simulink model "HANcoder_E407_TTA_Controller_v3"  (R2018b)
settings: Solver=FixedStepDiscrete  StartTime=0.0  StopTime=1  FixedStep=0.01  RelTol=1e-3
PreLoadFcn:
  | librarySetup
  | eval([bdroot,'_startup']) %Calling [modelName]_startup.m
values from neighbouring files (symbols this model uses):
  basic_cycle_duration_bc0 = TM_Reset_Board   + COMP_duration    (= 212)    [HANcoder_E407_TTA_Controller_v3_startup.m]
  basic_cycle_duration_bc1 = TM_Reset_Var_bc1 + COMP_duration    (= 288)    [HANcoder_E407_TTA_Controller_v3_startup.m]
  comm_delay_estimation1 = round(comm_delay_measured1*hardware_granularity/frequency_IRQ)    [HANcoder_E407_TTA_Controller_v3_startup.m]
  comm_delay_estimation2 = round(comm_delay_measured2*hardware_granularity/frequency_IRQ)    [HANcoder_E407_TTA_Controller_v3_startup.m]
  COMM_Period = 40    [HANcoder_E407_TTA_Controller_v3_startup.m]
  COMM_Phase1 = 5    [HANcoder_E407_TTA_Controller_v3_startup.m]
  COMM_Phase2 = 8    [HANcoder_E407_TTA_Controller_v3_startup.m]
  COMP_duration = 4    [HANcoder_E407_TTA_Controller_v3_startup.m]
  Controller1_Board = 1    [HANcoder_E407_TTA_Controller_v3_startup.m]
  Controller2_Board = 2    [HANcoder_E407_TTA_Controller_v3_startup.m]
  Controller3_Board = 3    [HANcoder_E407_TTA_Controller_v3_startup.m]
  delta_a_set = Simulink.Parameter    [HANcoder_E407_TTA_Controller_v3_startup.m]
  delta_f_set = Simulink.Parameter    [HANcoder_E407_TTA_Controller_v3_startup.m]
  delta_max = 1    [HANcoder_E407_TTA_Controller_v3_startup.m]
  delta_min = -1    [HANcoder_E407_TTA_Controller_v3_startup.m]
  delta_precision = 6    [HANcoder_E407_TTA_Controller_v3_startup.m]
  e_width = 0.1    [HANcoder_E407_TTA_Controller_v3_startup.m]
  frequency_IRQ = 100    [HANcoder_E407_TTA_Controller_v3_startup.m]
  HANtuneOverride = Simulink.Parameter    [HANcoder_E407_TTA_Controller_v3_startup.m]
  hardware_granularity = 1000000    [HANcoder_E407_TTA_Controller_v3_startup.m]
  I_a = 2.25    [HANcoder_E407_TTA_Controller_v3_startup.m]
  I_f = 2.25    [HANcoder_E407_TTA_Controller_v3_startup.m]
  idle_time_init = basic_cycle_duration_bc0 + basic_cycle_duration_bc1    (= 500)    [HANcoder_E407_TTA_Controller_v3_startup.m]
  Input_Gen_Board = 4    [HANcoder_E407_TTA_Controller_v3_startup.m]
  LA_Clock_Gr = 1    [HANcoder_E407_TTA_Controller_v3_startup.m]
  LA_COMM_dly = 0    [HANcoder_E407_TTA_Controller_v3_startup.m]
  LA_COMM_Err = 0    [HANcoder_E407_TTA_Controller_v3_startup.m]
  LA_E_Desync = 0    [HANcoder_E407_TTA_Controller_v3_startup.m]
  LA_MEX_Flag = 1    [HANcoder_E407_TTA_Controller_v3_startup.m]
  LA_Task_Act = 1    [HANcoder_E407_TTA_Controller_v3_startup.m]
  m_v = 100.0    (= 100)    [HANcoder_E407_TTA_Controller_v3_startup.m]
  Master_Role = 1    [HANcoder_E407_TTA_Controller_v3_startup.m]
  matrix_cycle_duration = basic_cycle_duration_bc0 + basic_cycle_duration_bc1    (= 500)    [HANcoder_E407_TTA_Controller_v3_startup.m]
  matrix_rows = 2    [HANcoder_E407_TTA_Controller_v3_startup.m]
  max_num_msgs_CAN1 = 2^Tx_bit_number-1    (= 7)    [HANcoder_E407_TTA_Controller_v3_startup.m]
  max_num_msgs_CAN2 = max_num_msgs_CAN1    (= 7)    [HANcoder_E407_TTA_Controller_v3_startup.m]
  OutControl1_ID = 23    [HANcoder_E407_TTA_Controller_v3_startup.m]
  OutControl2_ID = 24    [HANcoder_E407_TTA_Controller_v3_startup.m]
  OutEmulator_ID = 25    [HANcoder_E407_TTA_Controller_v3_startup.m]
  R_al = 0.10    (= 0.1)    [HANcoder_E407_TTA_Controller_v3_startup.m]
  R_ar = 0.10    (= 0.1)    [HANcoder_E407_TTA_Controller_v3_startup.m]
  R_fl = 0.10    (= 0.1)    [HANcoder_E407_TTA_Controller_v3_startup.m]
  R_fr = 0.10    (= 0.1)    [HANcoder_E407_TTA_Controller_v3_startup.m]
  script_run = Simulink.Parameter    [HANcoder_E407_TTA_Controller_v3_startup.m]
  SensorValues_ID = 22    [HANcoder_E407_TTA_Controller_v3_startup.m]
  SetValues_ID = 21    [HANcoder_E407_TTA_Controller_v3_startup.m]
  Slave_Role = 2    [HANcoder_E407_TTA_Controller_v3_startup.m]
  speed_k_d = Simulink.Parameter    [HANcoder_E407_TTA_Controller_v3_startup.m]
  speed_k_i = Simulink.Parameter    [HANcoder_E407_TTA_Controller_v3_startup.m]
  speed_k_p = Simulink.Parameter    [HANcoder_E407_TTA_Controller_v3_startup.m]
  speed_max = 10    [HANcoder_E407_TTA_Controller_v3_startup.m]
  speed_min = -10    [HANcoder_E407_TTA_Controller_v3_startup.m]
  speed_precision = 3    [HANcoder_E407_TTA_Controller_v3_startup.m]
  Sync_ID = 1    [HANcoder_E407_TTA_Controller_v3_startup.m]
  tau_max = 5    [HANcoder_E407_TTA_Controller_v3_startup.m]
  tau_min = -5    [HANcoder_E407_TTA_Controller_v3_startup.m]
  tau_range = abs(tau_max) + abs(tau_min)    [HANcoder_E407_TTA_Controller_v3_startup.m]
  theta_max = (speed_max/R_fr)*matrix_cycle_duration*frequency_IRQ/hardware_granularity    (= 5)    [HANcoder_E407_TTA_Controller_v3_startup.m]
  theta_min = (-1)*theta_max    (= -5)    [HANcoder_E407_TTA_Controller_v3_startup.m]
  theta_precision = 7-(fix(log2(theta_max))+1)    [HANcoder_E407_TTA_Controller_v3_startup.m]
  Tl_a = 0.6    [HANcoder_E407_TTA_Controller_v3_startup.m]
  Tl_f = 0.6    [HANcoder_E407_TTA_Controller_v3_startup.m]
  TM_Check_Output_Control1 = TM_COMM_Output_Control1 + COMM_duration    (= 188)    [HANcoder_E407_TTA_Controller_v3_startup.m]
  TM_Check_Output_Control2 = TM_COMM_Output_Control2 + COMM_duration    (= 232)    [HANcoder_E407_TTA_Controller_v3_startup.m]
  TM_Check_Output_Emulator = TM_COMM_Output_Emulator + COMM_duration    (= 280)    [HANcoder_E407_TTA_Controller_v3_startup.m]
  TM_Check_Sensor_Values = TM_COMM_Sensor_Values + COMM_duration    (= 132)    [HANcoder_E407_TTA_Controller_v3_startup.m]
  TM_Check_Set_Values = TM_COMM_Set_Values + COMM_duration    (= 88)    [HANcoder_E407_TTA_Controller_v3_startup.m]
  TM_Check_Sync = TM_COMM_Sync   + COMM_duration    (= 40)    [HANcoder_E407_TTA_Controller_v3_startup.m]
  TM_Check_TOuts = TM_Count_Vote3 + COMP_duration    (= 196)    [HANcoder_E407_TTA_Controller_v3_startup.m]
  TM_Check_Vote1 = TM_COMM_Vote1  + COMM_duration    (= 92)    [HANcoder_E407_TTA_Controller_v3_startup.m]
  TM_Check_Vote2 = TM_COMM_Vote2  + COMM_duration    (= 140)    [HANcoder_E407_TTA_Controller_v3_startup.m]
  TM_Check_Vote3 = TM_COMM_Vote3  + COMM_duration    (= 188)    [HANcoder_E407_TTA_Controller_v3_startup.m]
  TM_COMM_Output_Control1 = TM_Velocity + COMP_duration    (= 148)    [HANcoder_E407_TTA_Controller_v3_startup.m]
  TM_COMM_Output_Control2 = TM_Check_Output_Control1 + COMP_duration    (= 192)    [HANcoder_E407_TTA_Controller_v3_startup.m]
  TM_COMM_Output_Emulator = TM_TMR + COMP_duration    (= 240)    [HANcoder_E407_TTA_Controller_v3_startup.m]
  TM_COMM_Sensor_Values = TM_Check_Set_Values + COMP_duration    (= 92)    [HANcoder_E407_TTA_Controller_v3_startup.m]
  TM_COMM_Set_Values = TM_Update_LT + COMP_duration    (= 48)    [HANcoder_E407_TTA_Controller_v3_startup.m]
  TM_COMM_Sync = basic_cycle_start    (= 0)    [HANcoder_E407_TTA_Controller_v3_startup.m]
  TM_COMM_Vote1 = TM_Vote_Dec    + COMP_duration    (= 52)    [HANcoder_E407_TTA_Controller_v3_startup.m]
  TM_COMM_Vote2 = TM_Count_Vote1 + COMP_duration    (= 100)    [HANcoder_E407_TTA_Controller_v3_startup.m]
  TM_COMM_Vote3 = TM_Count_Vote2 + COMP_duration    (= 148)    [HANcoder_E407_TTA_Controller_v3_startup.m]
  TM_Count_Vote1 = TM_Check_Vote1 + COMP_duration    (= 96)    [HANcoder_E407_TTA_Controller_v3_startup.m]
  TM_Count_Vote2 = TM_Check_Vote2 + COMP_duration    (= 144)    [HANcoder_E407_TTA_Controller_v3_startup.m]
  TM_Count_Vote3 = TM_Check_Vote3 + COMP_duration    (= 192)    [HANcoder_E407_TTA_Controller_v3_startup.m]
  TM_Data_bc0 = TM_COMM_Sync    (= 0)    [HANcoder_E407_TTA_Controller_v3_startup.m]
  TM_Data_bc1 = TM_Data_bc0(1:3)    [HANcoder_E407_TTA_Controller_v3_startup.m]
  TM_New_Master = TM_Check_TOuts + COMP_duration    (= 200)    [HANcoder_E407_TTA_Controller_v3_startup.m]
  TM_Reset_Board = TM_Reset_Var   + COMP_duration    (= 208)    [HANcoder_E407_TTA_Controller_v3_startup.m]
  TM_Reset_Var = TM_New_Master  + COMP_duration    (= 204)    [HANcoder_E407_TTA_Controller_v3_startup.m]
  TM_Reset_Var_bc1 = TM_Check_Output_Emulator + COMP_duration    (= 284)    [HANcoder_E407_TTA_Controller_v3_startup.m]
  TM_Steer = TM_Check_Sensor_Values + COMP_duration    (= 136)    [HANcoder_E407_TTA_Controller_v3_startup.m]
  TM_TMR = TM_Check_Output_Control2 + COMP_duration    (= 236)    [HANcoder_E407_TTA_Controller_v3_startup.m]
  TM_Torque = TM_Steer + COMP_duration    (= 140)    [HANcoder_E407_TTA_Controller_v3_startup.m]
  TM_Type_bc0 = COMM    (= 0)    [HANcoder_E407_TTA_Controller_v3_startup.m]
  TM_Type_bc1 = TM_Type_bc0(1:3)    [HANcoder_E407_TTA_Controller_v3_startup.m]
  TM_Update_LT = TM_Check_Sync  + COMP_duration    (= 44)    [HANcoder_E407_TTA_Controller_v3_startup.m]
  TM_Velocity = TM_Torque + COMP_duration    (= 144)    [HANcoder_E407_TTA_Controller_v3_startup.m]
  TM_Vote_Dec = TM_Update_LT   + COMP_duration    (= 48)    [HANcoder_E407_TTA_Controller_v3_startup.m]
  torque_a_k_d = Simulink.Parameter    [HANcoder_E407_TTA_Controller_v3_startup.m]
  torque_a_k_i = Simulink.Parameter    [HANcoder_E407_TTA_Controller_v3_startup.m]
  torque_a_k_p = Simulink.Parameter    [HANcoder_E407_TTA_Controller_v3_startup.m]
  torque_f_k_d = Simulink.Parameter    [HANcoder_E407_TTA_Controller_v3_startup.m]
  torque_f_k_i = Simulink.Parameter    [HANcoder_E407_TTA_Controller_v3_startup.m]
  torque_f_k_p = Simulink.Parameter    [HANcoder_E407_TTA_Controller_v3_startup.m]
  torque_precision = 4    [HANcoder_E407_TTA_Controller_v3_startup.m]
  v_set = Simulink.Parameter    [HANcoder_E407_TTA_Controller_v3_startup.m]
  Vehicle_Em_Board = 5    [HANcoder_E407_TTA_Controller_v3_startup.m]
  Vote1_ID = 11    [HANcoder_E407_TTA_Controller_v3_startup.m]
  Vote2_ID = 12    [HANcoder_E407_TTA_Controller_v3_startup.m]
  Vote3_ID = 13    [HANcoder_E407_TTA_Controller_v3_startup.m]
undefined symbols (not defined in the file or in its folder): A0, A1, A2, A3, A4, CON2, CON4, D10, D12, D13, D8, D9
libraries: hdlsllib x352, HANcoder_STM32_Target x28, simulink x3, simulink_extras x1
(part 22 of 33)

== system HANcoder_E407_TTA_Controller_v3/HANcoder STM32 Target - E407-STM32 algorithm/Global Ticks Increment/CAN Management/Matrix Cycle Manager/Input Generator Matrix Cycle/input generator basic cycle 1/COMM Task - Set_Values/Reception substasks/RX buffers update ==
  note: Reset RX Buffer Flag
  note: Reception ID
      |    Sync Msg: 1
      |    Vote Node 1: 11
      |    Vote Node 2: 12
      |    Vote Node 3: 13
  note: Wait until new message
      | arrives
  note: Reset RX Buffer Flag
  note: Reception ID
      |    Sync Msg: 1
      |    Vote Node 1: 11
      |    Vote Node 2: 12
      |    Vote Node 3: 13
  note: Wait until new message
      | arrives
  note: Reset Rx buffers
  note: Reception end - Set RxID and Reset CAN buffer flags
  note: CAN1
  note: CAN2
  Rx_ID : Inport
  Enable : EnablePort
  Cast13 : DataTypeConversion  OutDataTypeStr=uint32
  Cast14 : DataTypeConversion  OutDataTypeStr=boolean
  Cast15 : DataTypeConversion  OutDataTypeStr=uint8
  Cast3 : DataTypeConversion  OutDataTypeStr=uint32
  Cast5 : DataTypeConversion  OutDataTypeStr=boolean
  Cast6 : DataTypeConversion  OutDataTypeStr=uint8
  Data Store Write : DataStoreWrite  DataStoreName=Msg_Rx
  Data Store Write11 : DataStoreWrite  DataStoreName=RxID_CAN2
  Data Store Write12 : DataStoreWrite  DataStoreName=Rx_State_CAN2
  Data Store Write2 : DataStoreWrite  DataStoreName=New_Msg_Ready_CAN1
  Data Store Write3 : DataStoreWrite  DataStoreName=new_msg_Rx
  Data Store Write6 : DataStoreWrite  DataStoreName=RxID_CAN1
  Data Store Write7 : DataStoreWrite  DataStoreName=Rx_State_CAN1
  Data Store Write9 : DataStoreWrite  DataStoreName=New_Msg_Ready_CAN2
  RESET1 : Constant  Value=0
  RESET2 : Constant  Value=0
  RESET_CAN1_new_buffer : Constant  Value=0
  RESET_CAN2_new_buffer : Constant  Value=0
  RESET_Msg_Rx : Constant  Value=0  OutDataTypeStr=Bus: msg_buffer_type
  RESET_new_msg_Rx : Constant  Value=0  OutDataTypeStr=boolean
  wires:
  Cast13/1 -> Data Store Write11/1
  Rx_ID/1 -> Cast3/1, Cast13/1
  RESET2/1 -> Cast14/1
  Cast14/1 -> Data Store Write9/1
  RESET_CAN2_new_buffer/1 -> Cast15/1
  Cast15/1 -> Data Store Write12/1
  Cast6/1 -> Data Store Write7/1
  RESET_CAN1_new_buffer/1 -> Cast6/1
  RESET_new_msg_Rx/1 -> Data Store Write3/1
  RESET_Msg_Rx/1 -> Data Store Write/1
  Cast5/1 -> Data Store Write2/1
  RESET1/1 -> Cast5/1
  Cast3/1 -> Data Store Write6/1

== system HANcoder_E407_TTA_Controller_v3/HANcoder STM32 Target - E407-STM32 algorithm/Global Ticks Increment/CAN Management/Matrix Cycle Manager/Input Generator Matrix Cycle/input generator basic cycle 1/COMM Task - Set_Values/Transmission subtasks/Check msg transmission CAN1 ==
  note: The TX buffers are updated one tick
      | before the message is sent
  note: A message should be sent during
      | this tick through CAN1
  note: In the next tick, a message will be
      | sent through CAN1
  Local Time : Inport
  Time Mark : Inport  Port=2
  Tx_ID : Inport  Port=3
  Value Domain Msg : Inport  Port=4
  Enable : EnablePort
  Constant11 : Constant  Value=0
  Constant22 : Constant
  Constant24 : Constant  Value=COMM_Phase1
  Constant27 : Constant  Value=COMM_Phase1
  Constant8 : Constant  Value=0
  Equal4 : RelationalOperator  Operator===  OutDataTypeStr=boolean  RndMeth=Simplest
  Equal7 : RelationalOperator  Operator===  OutDataTypeStr=boolean  RndMeth=Simplest
  Minus : Sum  Inputs=++-
  Minus1 : Sum  Inputs=+-
  Mod : Math  Operator=mod  SaturateOnIntegerOverflow=on
  Mod1 : Math  Operator=mod  SaturateOnIntegerOverflow=on
  TX buffer update CAN1 : Subsystem  Priority=20
  Send CAN1 : Outport  OutputWhenDisabled=reset  InitialOutput=0
  wires:
  Time Mark/1 -> Minus1/2, Minus/3
  Equal4/1 -> TX buffer update CAN1/Enable
  Constant22/1 -> Minus/2
  Local Time/1 -> Minus1/1, Minus/1
  Tx_ID/1 -> TX buffer update CAN1/1(Tx_ID)
  Mod1/1 -> Equal7/1
  Constant27/1 -> Mod1/2
  Minus/1 -> Mod/1
  Value Domain Msg/1 -> TX buffer update CAN1/2(Msg_Value_Data)
  Constant24/1 -> Mod/2
  Mod/1 -> Equal4/1
  Minus1/1 -> Mod1/1
  Constant11/1 -> Equal7/2
  Equal7/1 -> Send CAN1/1
  Constant8/1 -> Equal4/2

== system HANcoder_E407_TTA_Controller_v3/HANcoder STM32 Target - E407-STM32 algorithm/Global Ticks Increment/CAN Management/Matrix Cycle Manager/Input Generator Matrix Cycle/input generator basic cycle 1/COMM Task - Set_Values/Transmission subtasks/Check msg transmission CAN2 ==
  note: In the next tick, a message will be
      | sent through CAN2
  note: A message should be sent during
      | this tick through CAN2
  note: The TX buffers are updated one tick
      | before the message is sent
  Local Time : Inport
  Time Mark : Inport  Port=2
  Tx_ID : Inport  Port=3
  Value Domain Msg : Inport  Port=4
  Enable : EnablePort
  Constant11 : Constant  Value=0
  Constant22 : Constant
  Constant24 : Constant  Value=COMM_Phase2
  Constant27 : Constant  Value=COMM_Phase2
  Constant8 : Constant  Value=0
  Equal4 : RelationalOperator  Operator===  OutDataTypeStr=boolean  RndMeth=Simplest
  Equal7 : RelationalOperator  Operator===  OutDataTypeStr=boolean  RndMeth=Simplest
  Minus : Sum  Inputs=++-
  Minus1 : Sum  Inputs=+-
  Mod : Math  Operator=mod  SaturateOnIntegerOverflow=on
  Mod1 : Math  Operator=mod  SaturateOnIntegerOverflow=on
  TX buffer update CAN2 : Subsystem  Priority=20
  Send CAN2 : Outport  OutputWhenDisabled=reset  InitialOutput=0
  wires:
  Constant8/1 -> Equal4/2
  Equal7/1 -> Send CAN2/1
  Constant11/1 -> Equal7/2
  Minus1/1 -> Mod1/1
  Mod/1 -> Equal4/1
  Constant24/1 -> Mod/2
  Value Domain Msg/1 -> TX buffer update CAN2/2(Msg_Value_Data)
  Minus/1 -> Mod/1
  Constant27/1 -> Mod1/2
  Mod1/1 -> Equal7/1
  Tx_ID/1 -> TX buffer update CAN2/1(Tx_ID)
  Local Time/1 -> Minus/1, Minus1/1
  Constant22/1 -> Minus/2
  Equal4/1 -> TX buffer update CAN2/Enable
  Time Mark/1 -> Minus/3, Minus1/2

== system HANcoder_E407_TTA_Controller_v3/HANcoder STM32 Target - E407-STM32 algorithm/Global Ticks Increment/CAN Management/Matrix Cycle Manager/Input Generator Matrix Cycle/input generator basic cycle 1/COMM Task - Set_Values/Transmission subtasks/Msg_Value_Data_Encoded5 ==
  note: Value domain message encoding
      | <Warning!> The first buffer (from the top) is not used in transmission!
  Enable : EnablePort
  Bus Creator : BusCreator  Inputs=8  OutDataTypeStr=Bus: msg_buffer_type
  Constant : Constant  Value=0  OutDataTypeStr=uint8
  Constant1 : Constant  Value=delta_precision
  Constant10 : Constant  Value=delta_f_set
  Constant11 : Constant  Value=delta_a_set
  Constant12 : Constant  Value=v_set
  Constant2 : Constant  Value=delta_precision
  Constant3 : Constant  Value=speed_precision
  Constant4 : Constant  Value=delta_max
  Constant5 : Constant  Value=delta_min
  Constant6 : Constant  Value=delta_max
  Constant7 : Constant  Value=delta_min
  Constant8 : Constant  Value=speed_max
  Constant9 : Constant  Value=speed_min
  float2uint1 : Subsystem
  float2uint2 : Subsystem
  float2uint8 : Subsystem
  Value_domain_msg : Outport
  wires:
  Constant9/1 -> float2uint2/4(magnitude_min)
  Constant8/1 -> float2uint2/3(magnitude_max)
  Constant12/1 -> float2uint2/2(magnitude)
  Constant3/1 -> float2uint2/1(precision)
  Constant7/1 -> float2uint1/4(magnitude_min)
  Constant6/1 -> float2uint1/3(magnitude_max)
  Constant11/1 -> float2uint1/2(magnitude)
  Constant2/1 -> float2uint1/1(precision)
  Constant1/1 -> float2uint8/1(precision)
  Constant10/1 -> float2uint8/2(magnitude)
  Constant4/1 -> float2uint8/3(magnitude_max)
  Constant5/1 -> float2uint8/4(magnitude_min)
  float2uint2/1(coded) -> Bus Creator/4
  float2uint1/1(coded) -> Bus Creator/3
  float2uint8/1(coded) -> Bus Creator/2
  Constant/1 -> Bus Creator/6, Bus Creator/8, Bus Creator/7, Bus Creator/5, Bus Creator/1
  Bus Creator/1 -> Value_domain_msg/1

== system HANcoder_E407_TTA_Controller_v3/HANcoder STM32 Target - E407-STM32 algorithm/Global Ticks Increment/CAN Management/Matrix Cycle Manager/Input Generator Matrix Cycle/input generator basic cycle 1/COMM Task - Sync bc 1/Reception substasks/RX buffers update ==
  note: CAN2
  note: CAN1
  note: Reception end - Set RxID and Reset CAN buffer flags
  note: Reset Rx buffers
  note: Wait until new message
      | arrives
  note: Reception ID
      |    Sync Msg: 1
      |    Vote Node 1: 11
      |    Vote Node 2: 12
      |    Vote Node 3: 13
  note: Reset RX Buffer Flag
  note: Wait until new message
      | arrives
  note: Reception ID
      |    Sync Msg: 1
      |    Vote Node 1: 11
      |    Vote Node 2: 12
      |    Vote Node 3: 13
  note: Reset RX Buffer Flag
  Rx_ID : Inport
  Enable : EnablePort
  Cast13 : DataTypeConversion  OutDataTypeStr=uint32
  Cast14 : DataTypeConversion  OutDataTypeStr=boolean
  Cast15 : DataTypeConversion  OutDataTypeStr=uint8
  Cast3 : DataTypeConversion  OutDataTypeStr=uint32
  Cast5 : DataTypeConversion  OutDataTypeStr=boolean
  Cast6 : DataTypeConversion  OutDataTypeStr=uint8
  Data Store Write : DataStoreWrite  DataStoreName=Msg_Rx
  Data Store Write11 : DataStoreWrite  DataStoreName=RxID_CAN2
  Data Store Write12 : DataStoreWrite  DataStoreName=Rx_State_CAN2
  Data Store Write2 : DataStoreWrite  DataStoreName=New_Msg_Ready_CAN1
  Data Store Write3 : DataStoreWrite  DataStoreName=new_msg_Rx
  Data Store Write6 : DataStoreWrite  DataStoreName=RxID_CAN1
  Data Store Write7 : DataStoreWrite  DataStoreName=Rx_State_CAN1
  Data Store Write9 : DataStoreWrite  DataStoreName=New_Msg_Ready_CAN2
  RESET1 : Constant  Value=0
  RESET2 : Constant  Value=0
  RESET_CAN1_new_buffer : Constant  Value=0
  RESET_CAN2_new_buffer : Constant  Value=0
  RESET_Msg_Rx : Constant  Value=0  OutDataTypeStr=Bus: msg_buffer_type
  RESET_new_msg_Rx : Constant  Value=0  OutDataTypeStr=boolean
  wires:
  Cast3/1 -> Data Store Write6/1
  RESET1/1 -> Cast5/1
  Cast5/1 -> Data Store Write2/1
  RESET_Msg_Rx/1 -> Data Store Write/1
  RESET_new_msg_Rx/1 -> Data Store Write3/1
  RESET_CAN1_new_buffer/1 -> Cast6/1
  Cast6/1 -> Data Store Write7/1
  Cast15/1 -> Data Store Write12/1
  RESET_CAN2_new_buffer/1 -> Cast15/1
  Cast14/1 -> Data Store Write9/1
  RESET2/1 -> Cast14/1
  Rx_ID/1 -> Cast13/1, Cast3/1
  Cast13/1 -> Data Store Write11/1

== system HANcoder_E407_TTA_Controller_v3/HANcoder STM32 Target - E407-STM32 algorithm/Global Ticks Increment/CAN Management/Matrix Cycle Manager/Input Generator Matrix Cycle/input generator basic cycle 1/COMM Task - Sync bc 1/Transmission subtasks/Check msg transmission CAN1 ==
  note: In the next tick, a message will be
      | sent through CAN1
  note: A message should be sent during
      | this tick through CAN1
  note: The TX buffers are updated one tick
      | before the message is sent
  Local Time : Inport
  Time Mark : Inport  Port=2
  Tx_ID : Inport  Port=3
  Value Domain Msg : Inport  Port=4
  Enable : EnablePort
  Constant11 : Constant  Value=0
  Constant22 : Constant
  Constant24 : Constant  Value=COMM_Phase1
  Constant27 : Constant  Value=COMM_Phase1
  Constant8 : Constant  Value=0
  Equal4 : RelationalOperator  Operator===  OutDataTypeStr=boolean  RndMeth=Simplest
  Equal7 : RelationalOperator  Operator===  OutDataTypeStr=boolean  RndMeth=Simplest
  Minus : Sum  Inputs=++-
  Minus1 : Sum  Inputs=+-
  Mod : Math  Operator=mod  SaturateOnIntegerOverflow=on
  Mod1 : Math  Operator=mod  SaturateOnIntegerOverflow=on
  TX buffer update CAN1 : Subsystem  Priority=20
  Send CAN1 : Outport  OutputWhenDisabled=reset  InitialOutput=0
  wires:
  Constant8/1 -> Equal4/2
  Equal7/1 -> Send CAN1/1
  Constant11/1 -> Equal7/2
  Minus1/1 -> Mod1/1
  Mod/1 -> Equal4/1
  Constant24/1 -> Mod/2
  Value Domain Msg/1 -> TX buffer update CAN1/2(Msg_Value_Data)
  Minus/1 -> Mod/1
  Constant27/1 -> Mod1/2
  Mod1/1 -> Equal7/1
  Tx_ID/1 -> TX buffer update CAN1/1(Tx_ID)
  Local Time/1 -> Minus/1, Minus1/1
  Constant22/1 -> Minus/2
  Equal4/1 -> TX buffer update CAN1/Enable
  Time Mark/1 -> Minus/3, Minus1/2

== system HANcoder_E407_TTA_Controller_v3/HANcoder STM32 Target - E407-STM32 algorithm/Global Ticks Increment/CAN Management/Matrix Cycle Manager/Input Generator Matrix Cycle/input generator basic cycle 1/COMM Task - Sync bc 1/Transmission subtasks/Check msg transmission CAN2 ==
  note: The TX buffers are updated one tick
      | before the message is sent
  note: A message should be sent during
      | this tick through CAN2
  note: In the next tick, a message will be
      | sent through CAN2
  Local Time : Inport
  Time Mark : Inport  Port=2
  Tx_ID : Inport  Port=3
  Value Domain Msg : Inport  Port=4
  Enable : EnablePort
  Constant11 : Constant  Value=0
  Constant22 : Constant
  Constant24 : Constant  Value=COMM_Phase2
  Constant27 : Constant  Value=COMM_Phase2
  Constant8 : Constant  Value=0
  Equal4 : RelationalOperator  Operator===  OutDataTypeStr=boolean  RndMeth=Simplest
  Equal7 : RelationalOperator  Operator===  OutDataTypeStr=boolean  RndMeth=Simplest
  Minus : Sum  Inputs=++-
  Minus1 : Sum  Inputs=+-
  Mod : Math  Operator=mod  SaturateOnIntegerOverflow=on
  Mod1 : Math  Operator=mod  SaturateOnIntegerOverflow=on
  TX buffer update CAN2 : Subsystem  Priority=20
  Send CAN2 : Outport  OutputWhenDisabled=reset  InitialOutput=0
  wires:
  Time Mark/1 -> Minus1/2, Minus/3
  Equal4/1 -> TX buffer update CAN2/Enable
  Constant22/1 -> Minus/2
  Local Time/1 -> Minus1/1, Minus/1
  Tx_ID/1 -> TX buffer update CAN2/1(Tx_ID)
  Mod1/1 -> Equal7/1
  Constant27/1 -> Mod1/2
  Minus/1 -> Mod/1
  Value Domain Msg/1 -> TX buffer update CAN2/2(Msg_Value_Data)
  Constant24/1 -> Mod/2
  Mod/1 -> Equal4/1
  Minus1/1 -> Mod1/1
  Constant11/1 -> Equal7/2
  Equal7/1 -> Send CAN2/1
  Constant8/1 -> Equal4/2

== system HANcoder_E407_TTA_Controller_v3/HANcoder STM32 Target - E407-STM32 algorithm/Global Ticks Increment/CAN Management/Matrix Cycle Manager/Input Generator Matrix Cycle/input generator basic cycle 1/COMM Task - Sync bc 1/Transmission subtasks/Msg_Value_Data_Encoded ==
  note: Value domain message encoding
      | <Warning!> The first buffer (from the top) is not used in transmission!
  Enable : EnablePort
  Bus Creator : BusCreator  Inputs=8  OutDataTypeStr=Bus: msg_buffer_type
  Constant : Constant  Value=0  OutDataTypeStr=uint8
  Constant1 : Constant  Value=torque_precision
  Constant10 : Constant  Value=speed_max
  Constant11 : Constant  Value=speed_min
  Constant12 : Constant  Value=delta_max
  Constant13 : Constant  Value=delta_min
  Constant14 : Constant  Value=delta_max
  Constant15 : Constant  Value=delta_min
  Constant2 : Constant  Value=torque_precision
  Constant3 : Constant  Value=speed_precision
  Constant4 : Constant  Value=delta_precision
  Constant5 : Constant  Value=delta_precision
  Constant6 : Constant  Value=tau_max
  Constant7 : Constant  Value=tau_min
  Constant8 : Constant  Value=tau_max
  Constant9 : Constant  Value=tau_min
  Data Store Read33 : DataStoreRead  DataStoreName=speed_integral
  Data Store Read34 : DataStoreRead  DataStoreName=torque_ar_integral
  Data Store Read35 : DataStoreRead  DataStoreName=torque_fr_integral
  Data Store Read36 : DataStoreRead  DataStoreName=delta_a_est
  Data Store Read37 : DataStoreRead  DataStoreName=delta_f_est
  float2uint1 : Subsystem
  float2uint2 : Subsystem
  float2uint3 : Subsystem
  float2uint4 : Subsystem
  float2uint8 : Subsystem
  Value_domain_msg : Outport
  wires:
  Constant15/1 -> float2uint4/4(magnitude_min)
  Constant14/1 -> float2uint4/3(magnitude_max)
  Constant12/1 -> float2uint3/3(magnitude_max)
  Constant13/1 -> float2uint3/4(magnitude_min)
  Constant11/1 -> float2uint2/4(magnitude_min)
  Constant10/1 -> float2uint2/3(magnitude_max)
  Constant8/1 -> float2uint1/3(magnitude_max)
  Constant9/1 -> float2uint1/4(magnitude_min)
  Constant7/1 -> float2uint8/4(magnitude_min)
  Constant6/1 -> float2uint8/3(magnitude_max)
  float2uint4/1(coded) -> Bus Creator/6
  float2uint3/1(coded) -> Bus Creator/5
  float2uint2/1(coded) -> Bus Creator/4
  float2uint1/1(coded) -> Bus Creator/3
  float2uint8/1(coded) -> Bus Creator/2
  Data Store Read36/1 -> float2uint4/2(magnitude)
  Data Store Read37/1 -> float2uint3/2(magnitude)
  Data Store Read33/1 -> float2uint2/2(magnitude)
  Data Store Read34/1 -> float2uint1/2(magnitude)
  Data Store Read35/1 -> float2uint8/2(magnitude)
  Constant/1 -> Bus Creator/7, Bus Creator/8, Bus Creator/1
  Constant5/1 -> float2uint4/1(precision)
  Constant4/1 -> float2uint3/1(precision)
  Constant3/1 -> float2uint2/1(precision)
  Constant2/1 -> float2uint1/1(precision)
  Constant1/1 -> float2uint8/1(precision)
  Bus Creator/1 -> Value_domain_msg/1

== system HANcoder_E407_TTA_Controller_v3/HANcoder STM32 Target - E407-STM32 algorithm/Global Ticks Increment/CAN Management/Matrix Cycle Manager/Input Generator Matrix Cycle/input generator basic cycle 1/COMP Task - Sync bc1 check/Process_Messages/Demux message CAN1 and check coherence ==
  CAN1_Rx_msg : Inport  OutDataTypeStr=Bus: msg_buffer_type
  expected_basic_cycle : Inport  Port=2
  Enable : EnablePort
  Bus Creator : BusCreator  Inputs=8  OutDataTypeStr=Bus: msg_buffer_type
  Bus Selector : BusSelector  OutputSignals=Buffer_1,Buffer_2,Buffer_3,Buffer_4,Buffer_5,Buffer_6,Buffer_7,Buffer_8
  Constant : Constant  Value=0  OutDataTypeStr=uint8
  Equal1 : RelationalOperator  Operator===  OutDataTypeStr=boolean  RndMeth=Simplest
  Subsystem : Subsystem
  Terminator : Terminator
  msg_count>2_DEBUG : Subsystem
  CAN1_msg : Outport  OutDataTypeStr=Bus: msg_buffer_type
  Msg_Count_CAN1 : Outport  Port=2
  CAN1_msg_coherent : Outport  Port=3  OutputWhenDisabled=reset  InitialOutput=0
  wires:
  Constant/1 -> Bus Creator/1
  Bus Creator/1 -> CAN1_msg/1
  Subsystem/2(msg_count) -> Msg_Count_CAN1/1, msg_count>2_DEBUG/1(msg_c)
  Subsystem/1(basic_cycle) -> Equal1/1
  Bus Selector/1 -> Subsystem/1(Msg_Temporal_Data)  "<Buffer_1>"
  Bus Selector/4 -> Bus Creator/4  "<Buffer_4>"
  Bus Selector/8 -> Bus Creator/8  "<Buffer_8>"
  Bus Selector/7 -> Bus Creator/7  "<Buffer_7>"
  Bus Selector/5 -> Bus Creator/5  "<Buffer_5>"
  Bus Selector/6 -> Bus Creator/6  "<Buffer_6>"
  expected_basic_cycle/1 -> Equal1/2
  Equal1/1 -> CAN1_msg_coherent/1
  CAN1_Rx_msg/1 -> Bus Selector/1
  Bus Selector/3 -> Bus Creator/3  "<Buffer_3>"
  Bus Selector/2 -> Bus Creator/2  "<Buffer_2>"
  Subsystem/3(board_id) -> Terminator/1

== system HANcoder_E407_TTA_Controller_v3/HANcoder STM32 Target - E407-STM32 algorithm/Global Ticks Increment/CAN Management/Matrix Cycle Manager/Input Generator Matrix Cycle/input generator basic cycle 1/COMP Task - Sync bc1 check/Process_Messages/Demux message CAN1 and check coherence1 ==
  CAN2_Rx_msg : Inport  OutDataTypeStr=Bus: msg_buffer_type
  expected_basic_cycle : Inport  Port=2
  Enable : EnablePort
  Bus Creator : BusCreator  Inputs=8  OutDataTypeStr=Bus: msg_buffer_type
  Bus Selector : BusSelector  OutputSignals=Buffer_1,Buffer_2,Buffer_3,Buffer_4,Buffer_5,Buffer_6,Buffer_7,Buffer_8
  Constant : Constant  Value=0  OutDataTypeStr=uint8
  Equal1 : RelationalOperator  Operator===  OutDataTypeStr=boolean  RndMeth=Simplest
  Subsystem : Subsystem
  Terminator : Terminator
  msg_count>2_DEBUG : Subsystem
  CAN2_msg_coherent : Outport  OutputWhenDisabled=reset  InitialOutput=0
  Msg_Count_CAN2 : Outport  Port=2
  CAN2_msg : Outport  Port=3  OutDataTypeStr=Bus: msg_buffer_type
  wires:
  Constant/1 -> Bus Creator/1
  Bus Creator/1 -> CAN2_msg/1
  Subsystem/2(msg_count) -> Msg_Count_CAN2/1, msg_count>2_DEBUG/1(msg_c)
  Subsystem/1(basic_cycle) -> Equal1/1
  Bus Selector/1 -> Subsystem/1(Msg_Temporal_Data)  "<Buffer_1>"
  Bus Selector/4 -> Bus Creator/4  "<Buffer_4>"
  Bus Selector/8 -> Bus Creator/8  "<Buffer_8>"
  Bus Selector/7 -> Bus Creator/7  "<Buffer_7>"
  Bus Selector/5 -> Bus Creator/5  "<Buffer_5>"
  Bus Selector/6 -> Bus Creator/6  "<Buffer_6>"
  expected_basic_cycle/1 -> Equal1/2
  Equal1/1 -> CAN2_msg_coherent/1
  CAN2_Rx_msg/1 -> Bus Selector/1
  Bus Selector/3 -> Bus Creator/3  "<Buffer_3>"
  Bus Selector/2 -> Bus Creator/2  "<Buffer_2>"
  Subsystem/3(board_id) -> Terminator/1

== system HANcoder_E407_TTA_Controller_v3/HANcoder STM32 Target - E407-STM32 algorithm/Global Ticks Increment/CAN Management/Matrix Cycle Manager/Input Generator Matrix Cycle/input generator basic cycle 1/COMP Task - Sync bc1 check/Process_Messages/Desync calculation ==
  note: Estimation of the Local Time when the message was sent
  note: Desync CAN2
      | expected RX - Actual RX
  note: Desync CAN1
      | expected RX - Actual RX
  TM_COMM : Inport
  New_msg_CAN1 : Inport  Port=2
  msg_count_CAN1 : Inport  Port=3
  msg_count_CAN2 : Inport  Port=4
  Enable : EnablePort
  Constant : Constant  Value=COMM_Phase1
  Constant1 : Constant  Value=COMM_Phase2
  Data Store Read : DataStoreRead  DataStoreName=Msg_Rx_Ticks_CAN1
  Data Store Read1 : DataStoreRead  DataStoreName=Msg_Rx_Ticks_CAN2
  Data Store Write1 : DataStoreWrite  Priority=23  DataStoreName=Desync_Ticks
  Minus : Sum  Priority=21  Inputs=+-
  Minus1 : Sum  Priority=20  Inputs=+-
  Multiply : Product  Priority=10
  Multiply1 : Product  Priority=12
  Sum : Sum  Priority=11  Inputs=+++
  Sum1 : Sum  Priority=13  Inputs=+++
  Switch1 : Switch  Priority=22  Criteria=u2 > Threshold
  delay_estimation_1 : Constant  Value=comm_delay_estimation1
  delay_estimation_2 : Constant  Value=comm_delay_estimation2
  wires:
  TM_COMM/1 -> Sum1/2, Sum/2
  delay_estimation_1/1 -> Sum/3
  msg_count_CAN1/1 -> Multiply/2
  Switch1/1 -> Data Store Write1/1  "Desync_Sync_bc1_ing_s"
  Minus/1 -> Switch1/3
  Sum1/1 -> [expected_LT_CAN2]
  delay_estimation_2/1 -> Sum1/3
  Multiply1/1 -> Sum1/1
  [expected_LT_CAN1] -> Minus1/1
  [expected_LT_CAN2] -> Minus/1
  Data Store Read1/1 -> Minus/2
  Multiply/1 -> Sum/1
  Data Store Read/1 -> Minus1/2
  msg_count_CAN2/1 -> Multiply1/2
  Sum/1 -> [expected_LT_CAN1]
  Minus1/1 -> Switch1/1
  Constant/1 -> Multiply/1
  Constant1/1 -> Multiply1/1
  New_msg_CAN1/1 -> Switch1/2

== system HANcoder_E407_TTA_Controller_v3/HANcoder STM32 Target - E407-STM32 algorithm/Global Ticks Increment/CAN Management/Matrix Cycle Manager/Input Generator Matrix Cycle/input generator basic cycle 1/COMP Task - Update LT/Local Time Update/Desync_Negative ==
  note: Local Time Update
  note: Current Local Time correction
  note: Local time correction when Desync is negative
      | In this case the Local Time "goes back in time".
      | Previous tasks will not be activated because
      | sync_processed flag is alread set.
  Current_Local_Time : Inport
  Enable : EnablePort
  Cast : DataTypeConversion  Priority=13  OutDataTypeStr=uint16
  Data Store Read : DataStoreRead  Priority=11  DataStoreName=Desync_Ticks
  Data Store Write1 : DataStoreWrite  Priority=14  DataStoreName=Local_Ticks  DataStoreElements=Local_Ticks
  Minus : Sum  Priority=12
  wires:
  Current_Local_Time/1 -> Minus/1
  Cast/1 -> Data Store Write1/1
  Minus/1 -> Cast/1
  Data Store Read/1 -> Minus/2

== system HANcoder_E407_TTA_Controller_v3/HANcoder STM32 Target - E407-STM32 algorithm/Global Ticks Increment/CAN Management/Matrix Cycle Manager/Vehicle Emulator Matrix Cycle/vehicle emulator basic cycle 0/COMM Task - Sync bc 0/Reception substasks/RX buffers update ==
  note: Reset RX Buffer Flag
  note: Reception ID
      |    Sync Msg: 1
      |    Vote Node 1: 11
      |    Vote Node 2: 12
      |    Vote Node 3: 13
  note: Wait until new message
      | arrives
  note: Reset RX Buffer Flag
  note: Reception ID
      |    Sync Msg: 1
      |    Vote Node 1: 11
      |    Vote Node 2: 12
      |    Vote Node 3: 13
  note: Wait until new message
      | arrives
  note: Reset Rx buffers
  note: Reception end - Set RxID and Reset CAN buffer flags
  note: CAN1
  note: CAN2
  Rx_ID : Inport
  Enable : EnablePort
  Cast13 : DataTypeConversion  OutDataTypeStr=uint32
  Cast14 : DataTypeConversion  OutDataTypeStr=boolean
  Cast15 : DataTypeConversion  OutDataTypeStr=uint8
  Cast3 : DataTypeConversion  OutDataTypeStr=uint32
  Cast5 : DataTypeConversion  OutDataTypeStr=boolean
  Cast6 : DataTypeConversion  OutDataTypeStr=uint8
  Data Store Write : DataStoreWrite  DataStoreName=Msg_Rx
  Data Store Write11 : DataStoreWrite  DataStoreName=RxID_CAN2
  Data Store Write12 : DataStoreWrite  DataStoreName=Rx_State_CAN2
  Data Store Write2 : DataStoreWrite  DataStoreName=New_Msg_Ready_CAN1
  Data Store Write3 : DataStoreWrite  DataStoreName=new_msg_Rx
  Data Store Write6 : DataStoreWrite  DataStoreName=RxID_CAN1
  Data Store Write7 : DataStoreWrite  DataStoreName=Rx_State_CAN1
  Data Store Write9 : DataStoreWrite  DataStoreName=New_Msg_Ready_CAN2
  RESET1 : Constant  Value=0
  RESET2 : Constant  Value=0
  RESET_CAN1_new_buffer : Constant  Value=0
  RESET_CAN2_new_buffer : Constant  Value=0
  RESET_Msg_Rx : Constant  Value=0  OutDataTypeStr=Bus: msg_buffer_type
  RESET_new_msg_Rx : Constant  Value=0  OutDataTypeStr=boolean
  wires:
  Cast13/1 -> Data Store Write11/1
  Rx_ID/1 -> Cast3/1, Cast13/1
  RESET2/1 -> Cast14/1
  Cast14/1 -> Data Store Write9/1
  RESET_CAN2_new_buffer/1 -> Cast15/1
  Cast15/1 -> Data Store Write12/1
  Cast6/1 -> Data Store Write7/1
  RESET_CAN1_new_buffer/1 -> Cast6/1
  RESET_new_msg_Rx/1 -> Data Store Write3/1
  RESET_Msg_Rx/1 -> Data Store Write/1
  Cast5/1 -> Data Store Write2/1
  RESET1/1 -> Cast5/1
  Cast3/1 -> Data Store Write6/1

== system HANcoder_E407_TTA_Controller_v3/HANcoder STM32 Target - E407-STM32 algorithm/Global Ticks Increment/CAN Management/Matrix Cycle Manager/Vehicle Emulator Matrix Cycle/vehicle emulator basic cycle 0/COMM Task - Sync bc 0/Transmission subtasks/Check msg transmission CAN1 ==
  note: The TX buffers are updated one tick
      | before the message is sent
  note: A message should be sent during
      | this tick through CAN1
  note: In the next tick, a message will be
      | sent through CAN1
  Local Time : Inport
  Time Mark : Inport  Port=2
  Tx_ID : Inport  Port=3
  Value Domain Msg : Inport  Port=4
  Enable : EnablePort
  Constant11 : Constant  Value=0
  Constant22 : Constant
  Constant24 : Constant  Value=COMM_Phase1
  Constant27 : Constant  Value=COMM_Phase1
  Constant8 : Constant  Value=0
  Equal4 : RelationalOperator  Operator===  OutDataTypeStr=boolean  RndMeth=Simplest
  Equal7 : RelationalOperator  Operator===  OutDataTypeStr=boolean  RndMeth=Simplest
  Minus : Sum  Inputs=++-
  Minus1 : Sum  Inputs=+-
  Mod : Math  Operator=mod  SaturateOnIntegerOverflow=on
  Mod1 : Math  Operator=mod  SaturateOnIntegerOverflow=on
  TX buffer update CAN1 : Subsystem  Priority=20
  Send CAN1 : Outport  OutputWhenDisabled=reset  InitialOutput=0
  wires:
  Time Mark/1 -> Minus1/2, Minus/3
  Equal4/1 -> TX buffer update CAN1/Enable
  Constant22/1 -> Minus/2
  Local Time/1 -> Minus1/1, Minus/1
  Tx_ID/1 -> TX buffer update CAN1/1(Tx_ID)
  Mod1/1 -> Equal7/1
  Constant27/1 -> Mod1/2
  Minus/1 -> Mod/1
  Value Domain Msg/1 -> TX buffer update CAN1/2(Msg_Value_Data)
  Constant24/1 -> Mod/2
  Mod/1 -> Equal4/1
  Minus1/1 -> Mod1/1
  Constant11/1 -> Equal7/2
  Equal7/1 -> Send CAN1/1
  Constant8/1 -> Equal4/2

== system HANcoder_E407_TTA_Controller_v3/HANcoder STM32 Target - E407-STM32 algorithm/Global Ticks Increment/CAN Management/Matrix Cycle Manager/Vehicle Emulator Matrix Cycle/vehicle emulator basic cycle 0/COMM Task - Sync bc 0/Transmission subtasks/Check msg transmission CAN2 ==
  note: In the next tick, a message will be
      | sent through CAN2
  note: A message should be sent during
      | this tick through CAN2
  note: The TX buffers are updated one tick
      | before the message is sent
  Local Time : Inport
  Time Mark : Inport  Port=2
  Tx_ID : Inport  Port=3
  Value Domain Msg : Inport  Port=4
  Enable : EnablePort
  Constant11 : Constant  Value=0
  Constant22 : Constant
  Constant24 : Constant  Value=COMM_Phase2
  Constant27 : Constant  Value=COMM_Phase2
  Constant8 : Constant  Value=0
  Equal4 : RelationalOperator  Operator===  OutDataTypeStr=boolean  RndMeth=Simplest
  Equal7 : RelationalOperator  Operator===  OutDataTypeStr=boolean  RndMeth=Simplest
  Minus : Sum  Inputs=++-
  Minus1 : Sum  Inputs=+-
  Mod : Math  Operator=mod  SaturateOnIntegerOverflow=on
  Mod1 : Math  Operator=mod  SaturateOnIntegerOverflow=on
  TX buffer update CAN2 : Subsystem  Priority=20
  Send CAN2 : Outport  OutputWhenDisabled=reset  InitialOutput=0
  wires:
  Constant8/1 -> Equal4/2
  Equal7/1 -> Send CAN2/1
  Constant11/1 -> Equal7/2
  Minus1/1 -> Mod1/1
  Mod/1 -> Equal4/1
  Constant24/1 -> Mod/2
  Value Domain Msg/1 -> TX buffer update CAN2/2(Msg_Value_Data)
  Minus/1 -> Mod/1
  Constant27/1 -> Mod1/2
  Mod1/1 -> Equal7/1
  Tx_ID/1 -> TX buffer update CAN2/1(Tx_ID)
  Local Time/1 -> Minus/1, Minus1/1
  Constant22/1 -> Minus/2
  Equal4/1 -> TX buffer update CAN2/Enable
  Time Mark/1 -> Minus/3, Minus1/2

== system HANcoder_E407_TTA_Controller_v3/HANcoder STM32 Target - E407-STM32 algorithm/Global Ticks Increment/CAN Management/Matrix Cycle Manager/Vehicle Emulator Matrix Cycle/vehicle emulator basic cycle 0/COMM Task - Sync bc 0/Transmission subtasks/Msg_Value_Data_Encoded ==
  note: Value domain message encoding
      | <Warning!> The first buffer (from the top) is not used in transmission!
  Enable : EnablePort
  Bus Creator : BusCreator  Inputs=8  OutDataTypeStr=Bus: msg_buffer_type
  Constant : Constant  Value=0  OutDataTypeStr=uint8
  Constant1 : Constant  Value=torque_precision
  Constant10 : Constant  Value=speed_max
  Constant11 : Constant  Value=speed_min
  Constant12 : Constant  Value=delta_max
  Constant13 : Constant  Value=delta_min
  Constant14 : Constant  Value=delta_max
  Constant15 : Constant  Value=delta_min
  Constant2 : Constant  Value=torque_precision
  Constant3 : Constant  Value=speed_precision
  Constant4 : Constant  Value=delta_precision
  Constant5 : Constant  Value=delta_precision
  Constant6 : Constant  Value=tau_max
  Constant7 : Constant  Value=tau_min
  Constant8 : Constant  Value=tau_max
  Constant9 : Constant  Value=tau_min
  Data Store Read33 : DataStoreRead  DataStoreName=speed_integral
  Data Store Read34 : DataStoreRead  DataStoreName=torque_ar_integral
  Data Store Read35 : DataStoreRead  DataStoreName=torque_fr_integral
  Data Store Read36 : DataStoreRead  DataStoreName=delta_a_est
  Data Store Read37 : DataStoreRead  DataStoreName=delta_f_est
  float2uint1 : Subsystem
  float2uint2 : Subsystem
  float2uint3 : Subsystem
  float2uint4 : Subsystem
  float2uint8 : Subsystem
  Value_domain_msg : Outport
  wires:
  Bus Creator/1 -> Value_domain_msg/1
  Constant1/1 -> float2uint8/1(precision)
  Constant2/1 -> float2uint1/1(precision)
  Constant3/1 -> float2uint2/1(precision)
  Constant4/1 -> float2uint3/1(precision)
  Constant5/1 -> float2uint4/1(precision)
  Constant/1 -> Bus Creator/1, Bus Creator/8, Bus Creator/7
  Data Store Read35/1 -> float2uint8/2(magnitude)
  Data Store Read34/1 -> float2uint1/2(magnitude)
  Data Store Read33/1 -> float2uint2/2(magnitude)
  Data Store Read37/1 -> float2uint3/2(magnitude)
  Data Store Read36/1 -> float2uint4/2(magnitude)
  float2uint8/1(coded) -> Bus Creator/2
  float2uint1/1(coded) -> Bus Creator/3
  float2uint2/1(coded) -> Bus Creator/4
  float2uint3/1(coded) -> Bus Creator/5
  float2uint4/1(coded) -> Bus Creator/6
  Constant6/1 -> float2uint8/3(magnitude_max)
  Constant7/1 -> float2uint8/4(magnitude_min)
  Constant9/1 -> float2uint1/4(magnitude_min)
  Constant8/1 -> float2uint1/3(magnitude_max)
  Constant10/1 -> float2uint2/3(magnitude_max)
  Constant11/1 -> float2uint2/4(magnitude_min)
  Constant13/1 -> float2uint3/4(magnitude_min)
  Constant12/1 -> float2uint3/3(magnitude_max)
  Constant14/1 -> float2uint4/3(magnitude_max)
  Constant15/1 -> float2uint4/4(magnitude_min)

== system HANcoder_E407_TTA_Controller_v3/HANcoder STM32 Target - E407-STM32 algorithm/Global Ticks Increment/CAN Management/Matrix Cycle Manager/Vehicle Emulator Matrix Cycle/vehicle emulator basic cycle 0/COMP Task - Sync bc0 check/Process_Messages/Demux message CAN1 and check coherence ==
  CAN1_Rx_msg : Inport  OutDataTypeStr=Bus: msg_buffer_type
  expected_basic_cycle : Inport  Port=2
  Enable : EnablePort
  Bus Creator : BusCreator  Inputs=8  OutDataTypeStr=Bus: msg_buffer_type
  Bus Selector : BusSelector  OutputSignals=Buffer_1,Buffer_2,Buffer_3,Buffer_4,Buffer_5,Buffer_6,Buffer_7,Buffer_8
  Constant : Constant  Value=0  OutDataTypeStr=uint8
  Equal1 : RelationalOperator  Operator===  OutDataTypeStr=boolean  RndMeth=Simplest
  Subsystem : Subsystem
  Terminator : Terminator
  msg_count>2_DEBUG : Subsystem
  CAN1_msg : Outport  OutDataTypeStr=Bus: msg_buffer_type
  Msg_Count_CAN1 : Outport  Port=2
  CAN1_msg_coherent : Outport  Port=3  OutputWhenDisabled=reset  InitialOutput=0
  wires:
  Bus Selector/2 -> Bus Creator/2  "<Buffer_2>"
  Bus Selector/3 -> Bus Creator/3  "<Buffer_3>"
  CAN1_Rx_msg/1 -> Bus Selector/1
  Equal1/1 -> CAN1_msg_coherent/1
  expected_basic_cycle/1 -> Equal1/2
  Bus Selector/6 -> Bus Creator/6  "<Buffer_6>"
  Bus Selector/5 -> Bus Creator/5  "<Buffer_5>"
  Bus Selector/7 -> Bus Creator/7  "<Buffer_7>"
  Bus Selector/8 -> Bus Creator/8  "<Buffer_8>"
  Bus Selector/4 -> Bus Creator/4  "<Buffer_4>"
  Bus Selector/1 -> Subsystem/1(Msg_Temporal_Data)  "<Buffer_1>"
  Subsystem/1(basic_cycle) -> Equal1/1
  Subsystem/2(msg_count) -> msg_count>2_DEBUG/1(msg_c), Msg_Count_CAN1/1
  Bus Creator/1 -> CAN1_msg/1
  Constant/1 -> Bus Creator/1
  Subsystem/3(board_id) -> Terminator/1

== system HANcoder_E407_TTA_Controller_v3/HANcoder STM32 Target - E407-STM32 algorithm/Global Ticks Increment/CAN Management/Matrix Cycle Manager/Vehicle Emulator Matrix Cycle/vehicle emulator basic cycle 0/COMP Task - Sync bc0 check/Process_Messages/Demux message CAN1 and check coherence1 ==
  CAN2_Rx_msg : Inport  OutDataTypeStr=Bus: msg_buffer_type
  expected_basic_cycle : Inport  Port=2
  Enable : EnablePort
  Bus Creator : BusCreator  Inputs=8  OutDataTypeStr=Bus: msg_buffer_type
  Bus Selector : BusSelector  OutputSignals=Buffer_1,Buffer_2,Buffer_3,Buffer_4,Buffer_5,Buffer_6,Buffer_7,Buffer_8
  Constant : Constant  Value=0  OutDataTypeStr=uint8
  Equal1 : RelationalOperator  Operator===  OutDataTypeStr=boolean  RndMeth=Simplest
  Subsystem : Subsystem
  Terminator : Terminator
  msg_count>2_DEBUG : Subsystem
  CAN2_msg_coherent : Outport  OutputWhenDisabled=reset  InitialOutput=0
  Msg_Count_CAN2 : Outport  Port=2
  CAN2_msg : Outport  Port=3  OutDataTypeStr=Bus: msg_buffer_type
  wires:
  Bus Selector/2 -> Bus Creator/2  "<Buffer_2>"
  Bus Selector/3 -> Bus Creator/3  "<Buffer_3>"
  CAN2_Rx_msg/1 -> Bus Selector/1
  Equal1/1 -> CAN2_msg_coherent/1
  expected_basic_cycle/1 -> Equal1/2
  Bus Selector/6 -> Bus Creator/6  "<Buffer_6>"
  Bus Selector/5 -> Bus Creator/5  "<Buffer_5>"
  Bus Selector/7 -> Bus Creator/7  "<Buffer_7>"
  Bus Selector/8 -> Bus Creator/8  "<Buffer_8>"
  Bus Selector/4 -> Bus Creator/4  "<Buffer_4>"
  Bus Selector/1 -> Subsystem/1(Msg_Temporal_Data)  "<Buffer_1>"
  Subsystem/1(basic_cycle) -> Equal1/1
  Subsystem/2(msg_count) -> msg_count>2_DEBUG/1(msg_c), Msg_Count_CAN2/1
  Bus Creator/1 -> CAN2_msg/1
  Constant/1 -> Bus Creator/1
  Subsystem/3(board_id) -> Terminator/1

== system HANcoder_E407_TTA_Controller_v3/HANcoder STM32 Target - E407-STM32 algorithm/Global Ticks Increment/CAN Management/Matrix Cycle Manager/Vehicle Emulator Matrix Cycle/vehicle emulator basic cycle 0/COMP Task - Sync bc0 check/Process_Messages/Desync calculation ==
  note: Estimation of the Local Time when the message was sent
  note: Desync CAN2
      | expected RX - Actual RX
  note: Desync CAN1
      | expected RX - Actual RX
  TM_COMM : Inport
  New_msg_CAN1 : Inport  Port=2
  msg_count_CAN1 : Inport  Port=3
  msg_count_CAN2 : Inport  Port=4
  Enable : EnablePort
  Constant : Constant  Value=COMM_Phase1
  Constant1 : Constant  Value=COMM_Phase2
  Data Store Read : DataStoreRead  DataStoreName=Msg_Rx_Ticks_CAN1
  Data Store Read1 : DataStoreRead  DataStoreName=Msg_Rx_Ticks_CAN2
  Data Store Write1 : DataStoreWrite  Priority=23  DataStoreName=Desync_Ticks
  Minus : Sum  Priority=21  Inputs=+-
  Minus1 : Sum  Priority=20  Inputs=+-
  Multiply : Product  Priority=10
  Multiply1 : Product  Priority=12
  Sum : Sum  Priority=11  Inputs=+++
  Sum1 : Sum  Priority=13  Inputs=+++
  Switch1 : Switch  Priority=22  Criteria=u2 > Threshold
  delay_estimation_1 : Constant  Value=comm_delay_estimation1
  delay_estimation_2 : Constant  Value=comm_delay_estimation2
  wires:
  TM_COMM/1 -> Sum1/2, Sum/2
  delay_estimation_1/1 -> Sum/3
  msg_count_CAN1/1 -> Multiply/2
  Switch1/1 -> Data Store Write1/1  "Desync_Sync_bc0_vem_s"
  Minus/1 -> Switch1/3
  Sum1/1 -> [expected_LT_CAN2]
  delay_estimation_2/1 -> Sum1/3
  Multiply1/1 -> Sum1/1
  [expected_LT_CAN1] -> Minus1/1
  [expected_LT_CAN2] -> Minus/1
  Data Store Read1/1 -> Minus/2
  Multiply/1 -> Sum/1
  Data Store Read/1 -> Minus1/2
  msg_count_CAN2/1 -> Multiply1/2
  Sum/1 -> [expected_LT_CAN1]
  Minus1/1 -> Switch1/1
  Constant/1 -> Multiply/1
  Constant1/1 -> Multiply1/1
  New_msg_CAN1/1 -> Switch1/2

== system HANcoder_E407_TTA_Controller_v3/HANcoder STM32 Target - E407-STM32 algorithm/Global Ticks Increment/CAN Management/Matrix Cycle Manager/Vehicle Emulator Matrix Cycle/vehicle emulator basic cycle 0/COMP Task - Update LT/Local Time Update/Desync_Negative ==
  note: Local time correction when Desync is negative
      | In this case the Local Time "goes back in time".
      | Previous tasks will not be activated because
      | sync_processed flag is alread set.
  note: Current Local Time correction
  note: Local Time Update
  Current_Local_Time : Inport
  Enable : EnablePort
  Cast : DataTypeConversion  Priority=13  OutDataTypeStr=uint16
  Data Store Read : DataStoreRead  Priority=11  DataStoreName=Desync_Ticks
  Data Store Write1 : DataStoreWrite  Priority=14  DataStoreName=Local_Ticks  DataStoreElements=Local_Ticks
  Minus : Sum  Priority=12
  wires:
  Data Store Read/1 -> Minus/2
  Minus/1 -> Cast/1
  Cast/1 -> Data Store Write1/1
  Current_Local_Time/1 -> Minus/1

== system HANcoder_E407_TTA_Controller_v3/HANcoder STM32 Target - E407-STM32 algorithm/Global Ticks Increment/CAN Management/Matrix Cycle Manager/Vehicle Emulator Matrix Cycle/vehicle emulator basic cycle 0/COMP Task - Vehicle Emulator Calculate Angles/Vehicle Emulator Calculate Angles/Integral theta aft left ==
  note: Integral approximation:
  current_integral_value : Inport
  current_value : Inport  Port=2
  previous_value : Inport  Port=3
  incr_time : Inport  Port=4
  Gain : Gain  Gain=1/2
  Minus : Sum
  Minus2 : Sum
  Multiply : Product
  result : Outport
  wires:
  Minus/1 -> Gain/1
  Minus2/1 -> result/1
  Gain/1 -> Multiply/1
  current_integral_value/1 -> Minus2/1
  current_value/1 -> Minus/1
  previous_value/1 -> Minus/2
  incr_time/1 -> Multiply/2
  Multiply/1 -> Minus2/2

== system HANcoder_E407_TTA_Controller_v3/HANcoder STM32 Target - E407-STM32 algorithm/Global Ticks Increment/CAN Management/Matrix Cycle Manager/Vehicle Emulator Matrix Cycle/vehicle emulator basic cycle 0/COMP Task - Vehicle Emulator Calculate Angles/Vehicle Emulator Calculate Angles/Integral theta aft right ==
  note: Integral approximation:
  current_integral_value : Inport
  current_value : Inport  Port=2
  previous_value : Inport  Port=3
  incr_time : Inport  Port=4
  Gain : Gain  Gain=1/2
  Minus : Sum
  Minus2 : Sum
  Multiply : Product
  result : Outport
  wires:
  Multiply/1 -> Minus2/2
  incr_time/1 -> Multiply/2
  previous_value/1 -> Minus/2
  current_value/1 -> Minus/1
  current_integral_value/1 -> Minus2/1
  Gain/1 -> Multiply/1
  Minus2/1 -> result/1
  Minus/1 -> Gain/1

== system HANcoder_E407_TTA_Controller_v3/HANcoder STM32 Target - E407-STM32 algorithm/Global Ticks Increment/CAN Management/Matrix Cycle Manager/Vehicle Emulator Matrix Cycle/vehicle emulator basic cycle 0/COMP Task - Vehicle Emulator Calculate Angles/Vehicle Emulator Calculate Angles/Integral theta front left ==
  note: Integral approximation:
  current_integral_value : Inport
  current_value : Inport  Port=2
  previous_value : Inport  Port=3
  incr_time : Inport  Port=4
  Gain : Gain  Gain=1/2
  Minus : Sum
  Minus2 : Sum
  Multiply : Product
  result : Outport
  wires:
  Minus/1 -> Gain/1
  Minus2/1 -> result/1
  Gain/1 -> Multiply/1
  current_integral_value/1 -> Minus2/1
  current_value/1 -> Minus/1
  previous_value/1 -> Minus/2
  incr_time/1 -> Multiply/2
  Multiply/1 -> Minus2/2
